simulink model "Examen_junio_2020"  (R2022b)
settings: Solver=VariableStepAuto  StartTime=0.0  StopTime=80  MaxStep=0.01  RelTol=1e-3
libraries: slpidlib x1
settings Model: Creator=Pablo  LastModifiedBy=Pablo

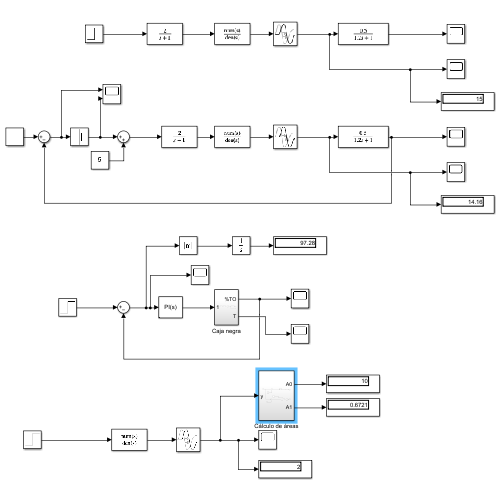
[thumbnail: Simulink's stored preview of the top-level diagram]
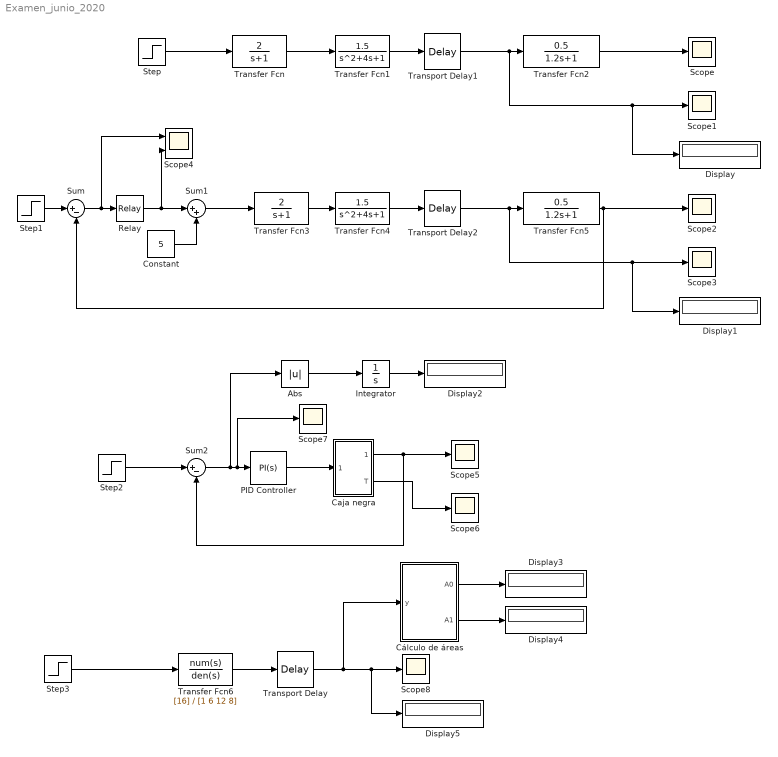
== system Examen_junio_2020 ==
  Abs : Abs  SaturateOnIntegerOverflow=off
  Caja negra : Subsystem
  Constant : Constant  Value=5
  Cálculo de áreas : Subsystem
  Display{,1..5} (6 alike) : Display
  Integrator : Integrator
  PID Controller : slpidlib/PID Controller  Controller=PI  Form=Ideal  TimeDomain=Continuous-time  UseExternalTs=off  SampleTime=-1  IntegratorMethod=Forward Euler  FilterMethod=Forward Euler  ControllerParametersSource=internal  P=0.964  I=1/8.13  UseKiTs=off  D=0  N=100  UseFilter=on  TunerSelectOption=Transfer Function Based (PID Tuner App)  InitialConditionSource=internal  InitialConditionForIntegrator=0  InitialConditionForFilter=0  DifferentiatorICPrevScaledInput=0  ExternalReset=none  TrackingMode=off  Kt=1  LimitOutput=off  SatLimitsSource=internal  UpperSaturationLimit=inf  LowerSaturationLimit=-inf  LinearizeAsGain=on  AntiWindupMode=none  Kb=1  LimitIntegrator=off  UpperIntegratorSaturationLimit=inf  LowerIntegratorSaturationLimit=-inf  POutMin=[]  POutMax=[]  IOutMin=[]  IOutMax=[]  DOutMin=[]  DOutMax=[]  NOutMin=[]  NOutMax=[]  SumOutMin=[]  SumOutMax=[]  SaturationOutMin=[]  SaturationOutMax=[]  PParamMin=[]  PParamMax=[]  IParamMin=[]  IParamMax=[]  DParamMin=[]  DParamMax=[]  NParamMin=[]  NParamMax=[]  KbParamMin=[]  KbParamMax=[]  KtParamMin=[]  KtParamMax=[]  KbOutMin=[]  KbOutMax=[]  KtOutMin=[]  KtOutMax=[]  IntegratorOutMin=[]  IntegratorOutMax=[]  FilterOutMin=[]  FilterOutMax=[]  SumI1OutMin=[]  SumI1OutMax=[]  SumI2OutMin=[]  SumI2OutMax=[]  SumI3OutMin=[]  SumI3OutMax=[]  SumI4OutMin=[]  SumI4OutMax=[]  SumDOutMin=[]  SumDOutMax=[]  DifferentiatorOutMin=[]  DifferentiatorOutMax=[]  FilterDiffOutCoefMin=[]  FilterDiffOutCoefMax=[]  ReciprocalOutMin=[]  ReciprocalOutMax=[]  SumDenOutMin=[]  SumDenOutMax=[]  SumNumOutMin=[]  SumNumOutMax=[]  DivideOutMin=[]  DivideOutMax=[]  UdiffTsProdOutMin=[]  UdiffTsProdOutMax=[]  NTsProdOutMin=[]  NTsProdOutMax=[]  UintegralTsProdOutMin=[]  UintegralTsProdOutMax=[]  UngainTsProdOutMin=[]  UngainTsProdOutMax=[]  ClampingZeroOutDataTypeStr=Inherit: Inherit via back propagation  ClampingZeroOutMin=[]  ClampingZeroOutMax=[]  FilterDenConstantOutDataTypeStr=Inherit: Inherit via back propagation  FilterDenConstantOutMin=[]  FilterDenConstantOutMax=[]  PCopyOutDataTypeStr=Inherit: Inherit via back propagation  PCopyOutMin=[]  PCopyOutMax=[]  NCopyOutDataTypeStr=Inherit: Inherit via back propagation  NCopyOutMin=[]  NCopyOutMax=[]  IntegratorContinuousStateAttributes=''  IntegratorStateMustResolveToSignalObject=off  IntegratorRTWStateStorageClass=Auto  FilterContinuousStateAttributes=''  FilterStateMustResolveToSignalObject=off  FilterRTWStateStorageClass=Auto  ParallelPVariant=Passthrough  IdealPVariant=InternalParameters  IVariant=InternalParameters  DVariant=Disabled  IntegratorVariant=Continuous  SatVariant=Disabled  AWVariant=Passthrough  PCopyVariant=Disabled  TRVariant=Disabled  FdbkBlocksVariant=Forward  IdealPFdbkVariant=Disabled  SatFdbkVariant=Disabled  DerivativeFilterVariant=Disabled  NVariant=Disabled  NCopyVariant=Disabled_SignalSpec  FilterICVariant=Disabled  IntegratorICVariant=InternalICs  ExternalResetVariant=Disabled  TRSumVariant=Passthrough  SumFdbkVariant=Disabled  SumVariant=Sum_PI  TsampFilterVariant=InternalTs  TsampNgainVariant=Passthrough  TsampIntegralVariant=Passthrough  ExternalSaturationOutDataTypeStr=Inherit: Same as second input
  Relay : Relay  OffOutputValue=-1
  Scope{,1..3,5..8} (8 alike) : Scope
  Scope4 : Scope  NumInputPorts=2
  Step : Step  After=5  SampleTime=0
  Step1 : Step  After=7.5  SampleTime=0
  Step2 : Step  Time=0  After=15  SampleTime=0
  Step3 : Step  SampleTime=0
  Sum : Sum  Inputs=|+-
  Sum1 : Sum  Inputs=|++
  Sum2 : Sum  Inputs=|+-
  Transfer Fcn : TransferFcn  Numerator=[2]  Denominator=[1 1]
  Transfer Fcn1 : TransferFcn  Numerator=[1.5]  Denominator=[1 4 1]
  Transfer Fcn2 : TransferFcn  Numerator=[0.5]  Denominator=[1.2 1]
  Transfer Fcn3 : TransferFcn  Numerator=[2]  Denominator=[1 1]
  Transfer Fcn4 : TransferFcn  Numerator=[1.5]  Denominator=[1 4 1]
  Transfer Fcn5 : TransferFcn  Numerator=[0.5]  Denominator=[1.2 1]
  Transfer Fcn6 : TransferFcn  Numerator=[16]  Denominator=[1 6 12 8]
  Transport Delay : TransportDelay  DelayTime=2.5
  Transport Delay1 : TransportDelay
  Transport Delay2 : TransportDelay
  wires:
  Transfer Fcn1/1 -> Transport Delay1/1
  Transport Delay1/1 -> Display/1, Scope1/1, Transfer Fcn2/1
  Transfer Fcn/1 -> Transfer Fcn1/1
  Transfer Fcn2/1 -> Scope/1
  Step/1 -> Transfer Fcn/1
  Transport Delay2/1 -> Display1/1, Scope3/1, Transfer Fcn5/1
  Transfer Fcn4/1 -> Transport Delay2/1
  Transfer Fcn5/1 -> Sum/2, Scope2/1
  Transfer Fcn3/1 -> Transfer Fcn4/1
  Sum/1 -> Scope4/1, Relay/1
  Step1/1 -> Sum/1
  Sum1/1 -> Transfer Fcn3/1
  Relay/1 -> Scope4/2, Sum1/1
  Constant/1 -> Sum1/2
  Caja negra/1(%TO) -> Sum2/2, Scope5/1
  Caja negra/2(T) -> Scope6/1
  Sum2/1 -> Abs/1, Scope7/1, PID Controller/1
  PID Controller/1 -> Caja negra/1(In1)
  Step2/1 -> Sum2/1
  Abs/1 -> Integrator/1
  Integrator/1 -> Display2/1
  Transfer Fcn6/1 -> Transport Delay/1
  Transport Delay/1 -> Cálculo de áreas/1(y), Display5/1, Scope8/1
  Cálculo de áreas/1(A0) -> Display3/1
  Cálculo de áreas/2(A1) -> Display4/1
  Step3/1 -> Transfer Fcn6/1

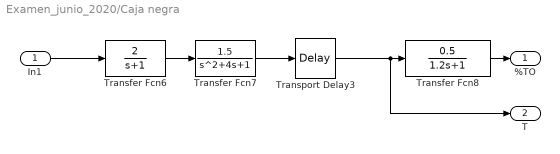
== system Examen_junio_2020/Caja negra ==
  In1 : Inport
  Transfer Fcn6 : TransferFcn  Numerator=[2]  Denominator=[1 1]
  Transfer Fcn7 : TransferFcn  Numerator=[1.5]  Denominator=[1 4 1]
  Transfer Fcn8 : TransferFcn  Numerator=[0.5]  Denominator=[1.2 1]
  Transport Delay3 : TransportDelay
  %TO : Outport
  T : Outport  Port=2
  wires:
  Transport Delay3/1 -> T/1, Transfer Fcn8/1
  Transfer Fcn6/1 -> Transfer Fcn7/1
  In1/1 -> Transfer Fcn6/1
  Transfer Fcn7/1 -> Transport Delay3/1
  Transfer Fcn8/1 -> %TO/1

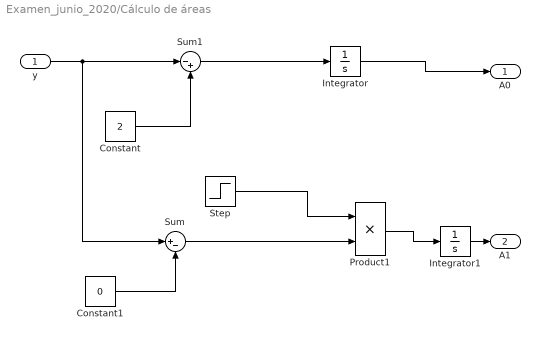
== system Examen_junio_2020/Cálculo de áreas ==
  y : Inport
  Constant : Constant  Value=2
  Constant1 : Constant  Value=0
  Integrator : Integrator
  Integrator1 : Integrator
  Product1 : Product
  Step : Step  Time=5  Before=1  After=0  SampleTime=0
  Sum : Sum  Inputs=|+-
  Sum1 : Sum  Inputs=|-+
  A0 : Outport
  A1 : Outport  Port=2
  wires:
  Step/1 -> Product1/1
  Sum/1 -> Product1/2
  Integrator1/1 -> A1/1
  Product1/1 -> Integrator1/1
  Sum1/1 -> Integrator/1
  Constant/1 -> Sum1/2
  Constant1/1 -> Sum/2
  Integrator/1 -> A0/1
  y/1 -> Sum/1, Sum1/1
